simulink model "sampleModel41"  (R2021b)
settings: Solver=VariableStepAuto  StartTime=0.0  StopTime=10.0  RelTol=1e-3
undefined symbols (not defined in the file or in its folder): magnitude
libraries: simulink x4
settings Model: Creator=user  LastModifiedBy=user

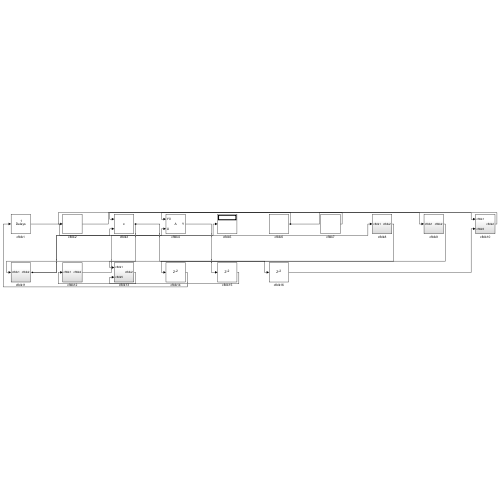
[thumbnail: Simulink's stored preview of the top-level diagram]
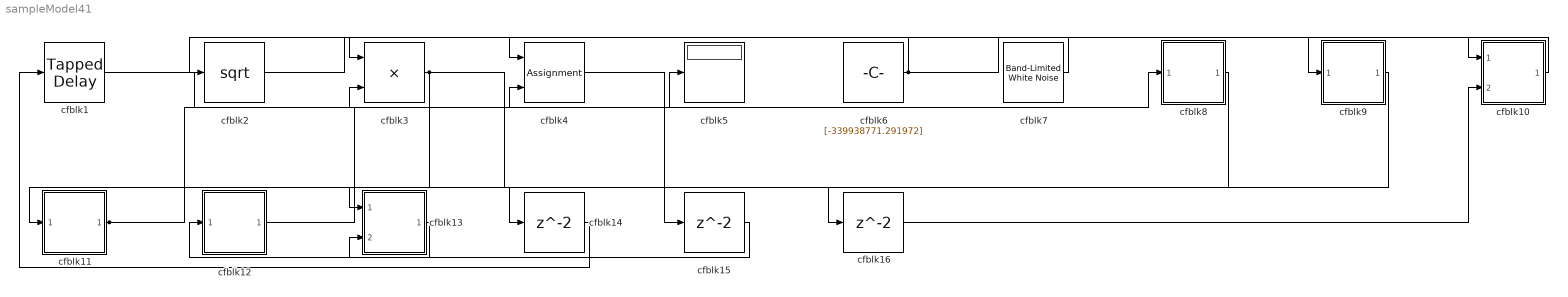
== system sampleModel41 ==
  cfblk1 : simulink/Discrete/Tapped Delay  vinit=0.0  samptime=-1  NumDelays=1  DelayOrder=Oldest  includeCurrent=off
  cfblk10 : Subsystem
  cfblk11 : Subsystem
  cfblk12 : Subsystem
  cfblk13 : Subsystem
  cfblk14 : Delay  SampleTime=1
  cfblk15 : Delay  SampleTime=1
  cfblk16 : Delay  SampleTime=1
  cfblk2 : Sqrt  SaturateOnIntegerOverflow=on
  cfblk3 : Product  Inputs=**
  cfblk4 : Assignment  DiagnosticForDimensions=Warning  IndexOptions=Index vector (dialog)  Indices=1  OutputSizes=1
  cfblk5 : Display
  cfblk6 : Constant  Value=[-339938771.291972]  SampleTime=1
  cfblk7 : simulink/Sources/Band-Limited White Noise  Cov=[7245869006.540229]  Ts=0.1  seed=[5849549834.000000]
  cfblk8 : Subsystem
  cfblk9 : Subsystem
  wires:
  cfblk9/1(cfblk2) -> cfblk11/1(cfblk1)
  cfblk13/1(cfblk2) -> cfblk12/1(cfblk1)
  cfblk10/1(cfblk2) -> cfblk3/1
  cfblk1/1 -> cfblk8/1(cfblk1)
  cfblk6/1 -> cfblk2/1, cfblk9/1(cfblk1)
  cfblk7/1 -> cfblk4/1
  cfblk2/1 -> cfblk10/1(cfblk1)
  cfblk12/1(cfblk2) -> cfblk4/2
  cfblk3/1 -> cfblk13/1(cfblk1), cfblk16/1
  cfblk11/1(cfblk2) -> cfblk5/1, cfblk3/2
  cfblk8/1(cfblk2) -> cfblk14/1
  cfblk14/1 -> cfblk1/1
  cfblk4/1 -> cfblk15/1
  cfblk15/1 -> cfblk13/2(cfblk5)
  cfblk16/1 -> cfblk10/2(cfblk5)

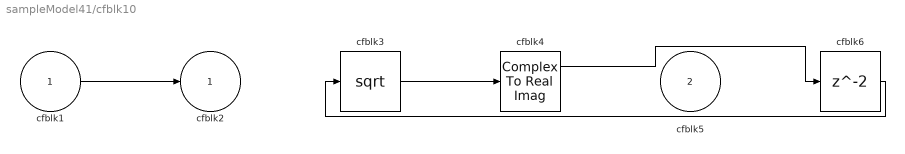
== system sampleModel41/cfblk10 ==
  cfblk1 : Inport
  cfblk5 : Inport  Port=2
  cfblk3 : Sqrt  SaturateOnIntegerOverflow=on
  cfblk4 : ComplexToRealImag
  cfblk6 : Delay  SampleTime=1
  cfblk2 : Outport
  wires:
  cfblk1/1 -> cfblk2/1
  cfblk3/1 -> cfblk4/1
  cfblk4/1 -> cfblk6/1
  cfblk6/1 -> cfblk3/1

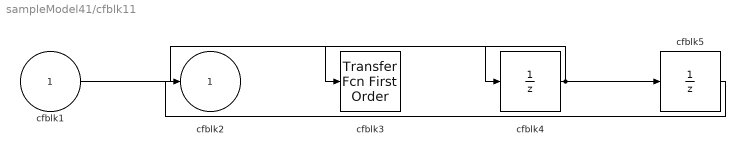
== system sampleModel41/cfblk11 ==
  cfblk1 : Inport
  cfblk3 : simulink/Discrete/Transfer Fcn First Order  PoleZ=0.95  ICPrevOutput=0.0  DoSatur=off
  cfblk4 : UnitDelay  HasFrameUpgradeWarning=on
  cfblk5 : UnitDelay  HasFrameUpgradeWarning=on
  cfblk2 : Outport
  wires:
  cfblk4/1 -> cfblk5/1, cfblk3/1
  cfblk1/1 -> cfblk4/1
  cfblk5/1 -> cfblk2/1

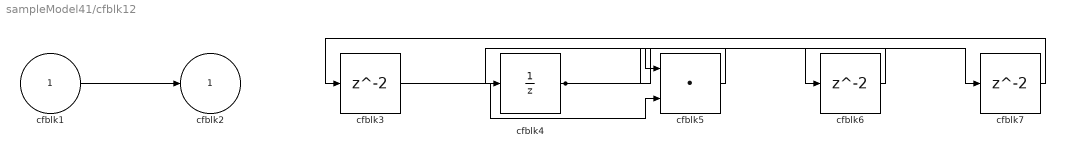
== system sampleModel41/cfblk12 ==
  cfblk1 : Inport
  cfblk3 : Delay  SampleTime=1
  cfblk4 : UnitDelay  HasFrameUpgradeWarning=on
  cfblk5 : DotProduct  InputSameDT=on  OutDataTypeStr=Inherit: Inherit via internal rule
  cfblk6 : Delay  SampleTime=1
  cfblk7 : Delay  SampleTime=1
  cfblk2 : Outport
  wires:
  cfblk4/1 -> cfblk6/1, cfblk7/1
  cfblk3/1 -> cfblk5/2
  cfblk5/1 -> cfblk4/1
  cfblk1/1 -> cfblk2/1
  cfblk6/1 -> cfblk5/1
  cfblk7/1 -> cfblk3/1

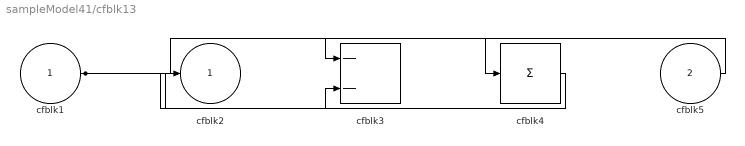
== system sampleModel41/cfblk13 ==
  cfblk1 : Inport
  cfblk5 : Inport  Port=2
  cfblk3 : Sum  Inputs=--
  cfblk4 : Sum  Inputs=+
  cfblk2 : Outport
  wires:
  cfblk1/1 -> cfblk4/1, cfblk3/2
  cfblk4/1 -> cfblk2/1
  cfblk5/1 -> cfblk3/1

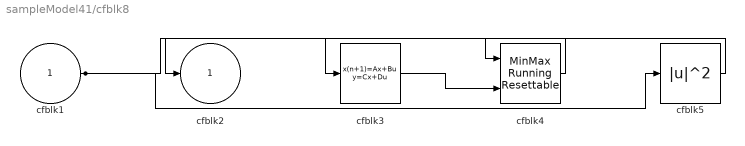
== system sampleModel41/cfblk8 ==
  cfblk1 : Inport
  cfblk3 : DiscreteStateSpace
  cfblk4 : simulink/Math Operations/MinMax Running Resettable  Function=min  vinit=0.0
  cfblk5 : Math  Operator=magnitude^2  SaturateOnIntegerOverflow=on
  cfblk2 : Outport
  wires:
  cfblk4/1 -> cfblk2/1
  cfblk1/1 -> cfblk5/1, cfblk3/1
  cfblk5/1 -> cfblk4/1
  cfblk3/1 -> cfblk4/2

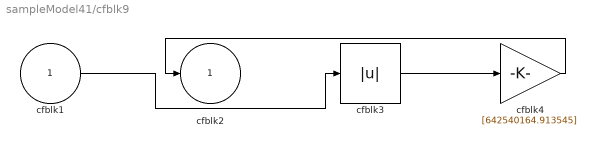
== system sampleModel41/cfblk9 ==
  cfblk1 : Inport
  cfblk3 : Abs
  cfblk4 : Gain  Gain=[642540164.913545]
  cfblk2 : Outport
  wires:
  cfblk3/1 -> cfblk4/1
  cfblk4/1 -> cfblk2/1
  cfblk1/1 -> cfblk3/1
